simulink model "AGTF30SysDyn_PExPIn"  (R2023b)
settings: Solver=ode4  StartTime=0.0  StopTime=MWS.In.tend  FixedStep=MWS.In.Ts  RelTol=1e-3  EnableMultiTasking=on
model workspace: external: MAT-File (data not in the file)
values from neighbouring files (symbols this model uses):
  MWS = setup_initialize(MWS,startPt,SSsolverSP)    [Setup_Simulation.m]    (also in run_AGTF30e_script.m = Setup_Simulation(inputMethod,MWS.In,filename,Mdl,SSsolverSP))
undefined symbols (not defined in the file or in its folder): DiscIntNeverNeededParam
libraries: simulink x32, Lib_Solve_ModelSource_TMATS x28, Lib_EMTAT x27, Lib_Cntrl_FirstOrderSensor_TMATS x19, Lib_Cntrl_FirstOrderActuator_TMATS x2, Lib_Cntrl_LimitSelect_TMATS x2, Lib_Solve_OuterLoopIntegrator_TMATS x2, Lib_Cntrl_CorrectedSpeed_TMATS x1, Lib_Solve_IterNRSolverJC_TMATS x1, slpidlib x1
(part 2 of 8)

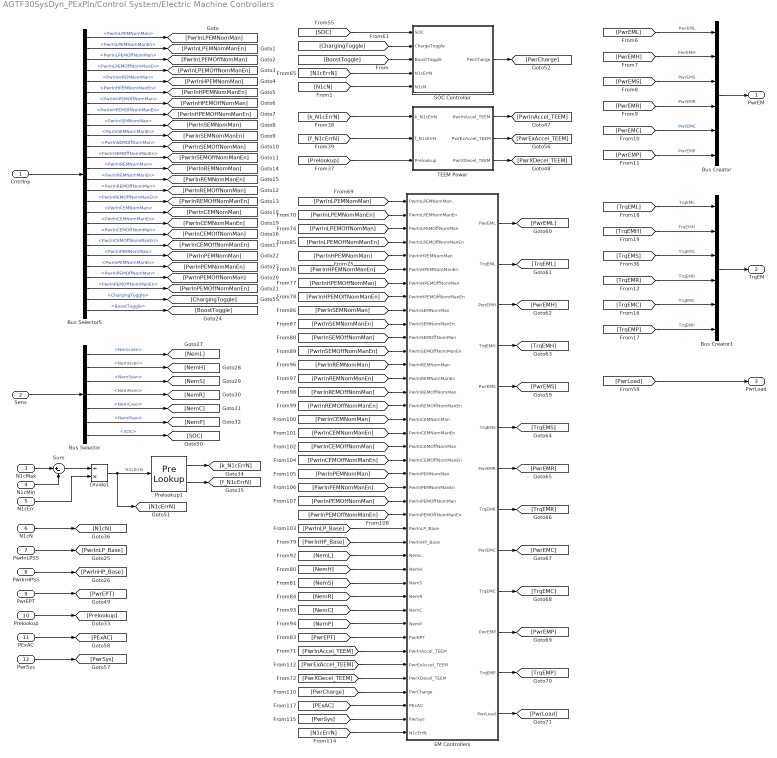
== system AGTF30SysDyn_PExPIn/Control System/Electric Machine Controllers ==
  CntrlInp : Inport
  Sens : Inport  Port=2
  N1cMax : Inport  Port=3
  N1cMin : Inport  Port=4
  N1cErr : Inport  Port=5
  N1cN : Inport  Port=6
  PwrInLPSS : Inport  Port=7
  PwrInHPSS : Inport  Port=8
  PwrEPT : Inport  Port=9
  Prelookup : Inport  Port=10
  PExAC : Inport  Port=11
  PwrSys : Inport  Port=12
  Bus Creator : BusCreator  Inputs=6
  Bus Creator1 : BusCreator  Inputs=6
  Bus Selector : BusSelector  OutputSignals=N.NemLsen,N.NemHsen,N.NemSsen,N.NemRsen,N.NemCsen,N.NemPsen,SOC
  Bus Selector5 : BusSelector  OutputSignals=ManualOp.PwrInLPEMNomMan,ManualOp.PwrInLPEMNomManEn,ManualOp.PwrInLPEMOffNomMan,ManualOp.PwrInLPEMOffNomManEn,ManualOp.PwrInHPEMNomMan,ManualOp.PwrInHPEMNomManEn,ManualOp.PwrInHPEMOffNomMan,ManualOp.PwrInHPEMOffNomManEn,ManualOp.PwrInSEMNomMan,ManualOp.PwrInSEMNomManEn,ManualOp.PwrInSEMOffNomMan,ManualOp.PwrInSEMOffNomManEn,ManualOp.PwrInREMNomMan,ManualOp.PwrInREMNomManEn,ManualOp.PwrInREMOffNomMan,ManualOp.PwrInREMOffNomManEn,ManualOp.PwrInCEMNomMan,ManualOp.PwrInCEMNomManEn,ManualOp.PwrInCEMOffNomMan,ManualOp.PwrInCEMOffNomManEn,ManualOp.PwrInPEMNomMan,ManualOp.PwrInPEMNomManEn,ManualOp.PwrInPEMOffNomMan,ManualOp.PwrInPEMOffNomManEn,PilotCmd.ChargingToggle,PilotCmd.BoostToggle
  Divide1 : Product  Inputs=/*
  EM Controllers : Subsystem  Variant=on
  Prelookup1 : PreLookup  BreakpointsData=MWS.Cntrl.TEEM.N1cErrN_vec  ExtrapMethod=Linear
  SOC Controller : Subsystem
  Sum : Sum  Inputs=|+-
  TEEM Power : Subsystem
  PwrEM : Outport
  TrqEM : Outport  Port=2
  PwrLoad : Outport  Port=3
  wires:
  Bus Selector5/19 -> [PwrInCEMOffNomMan]  "<PwrInCEMOffNomMan>"
  Sum/1 -> Divide1/1
  Bus Selector5/10 -> [PwrInSEMNomManEn]  "<PwrInSEMNomManEn>"
  Bus Selector5/4 -> [PwrInLPEMOffNomManEn]  "<PwrInLPEMOffNomManEn>"
  Bus Selector5/13 -> [PwrInREMNomMan]  "<PwrInREMNomMan>"
  Bus Selector5/24 -> [PwrInPEMOffNomManEn]  "<PwrInPEMOffNomManEn>"
  Bus Selector5/18 -> [PwrInCEMNomManEn]  "<PwrInCEMNomManEn>"
  Bus Selector5/20 -> [PwrInCEMOffNomManEn]  "<PwrInCEMOffNomManEn>"
  Bus Selector5/15 -> [PwrInREMOffNomMan]  "<PwrInREMOffNomMan>"
  Bus Selector5/17 -> [PwrInCEMNomMan]  "<PwrInCEMNomMan>"
  Bus Selector5/1 -> [PwrInLPEMNomMan]  "<PwrInLPEMNomMan>"
  Bus Selector5/21 -> [PwrInPEMNomMan]  "<PwrInPEMNomMan>"
  Bus Selector5/23 -> [PwrInPEMOffNomMan]  "<PwrInPEMOffNomMan>"
  Bus Selector5/11 -> [PwrInSEMOffNomMan]  "<PwrInSEMOffNomMan>"
  Bus Selector5/22 -> [PwrInPEMNomManEn]  "<PwrInPEMNomManEn>"
  N1cErr/1 -> Divide1/2
  Bus Selector5/6 -> [PwrInHPEMNomManEn]  "<PwrInHPEMNomManEn>"
  PwrInLPSS/1 -> [PwrInLP_Base]
  N1cMax/1 -> Sum/1
  Bus Selector5/9 -> [PwrInSEMNomMan]  "<PwrInSEMNomMan>"
  Bus Selector5/7 -> [PwrInHPEMOffNomMan]  "<PwrInHPEMOffNomMan>"
  Bus Selector5/8 -> [PwrInHPEMOffNomManEn]  "<PwrInHPEMOffNomManEn>"
  Bus Selector5/5 -> [PwrInHPEMNomMan]  "<PwrInHPEMNomMan>"
  Bus Selector5/3 -> [PwrInLPEMOffNomMan]  "<PwrInLPEMOffNomMan>"
  Bus Selector5/14 -> [PwrInREMNomManEn]  "<PwrInREMNomManEn>"
  Bus Selector5/12 -> [PwrInSEMOffNomManEn]  "<PwrInSEMOffNomManEn>"
  Bus Selector5/16 -> [PwrInREMOffNomManEn]  "<PwrInREMOffNomManEn>"
  CntrlInp/1 -> Bus Selector5/1
  Bus Selector5/2 -> [PwrInLPEMNomManEn]  "<PwrInLPEMNomManEn>"
  N1cMin/1 -> Sum/2
  Divide1/1 -> [N1cErrN], Prelookup1/1  "N1cErrN"
  PwrInHPSS/1 -> [PwrInHP_Base]
  Sens/1 -> Bus Selector/1
  Bus Selector/1 -> [NemL]  "<NemLsen>"
  Bus Selector/2 -> [NemH]  "<NemHsen>"
  Bus Selector/3 -> [NemS]  "<NemSsen>"
  Bus Selector/4 -> [NemR]  "<NemRsen>"
  Bus Selector/5 -> [NemC]  "<NemCsen>"
  Bus Selector/6 -> [NemP]  "<NemPsen>"
  Bus Creator/1 -> PwrEM/1
  [PwrEML] -> Bus Creator/1  "PwrEML"
  [PwrEMH] -> Bus Creator/2  "PwrEMH"
  [PwrEMS] -> Bus Creator/3  "PwrEMS"
  [PwrEMR] -> Bus Creator/4  "PwrEMR"
  [PwrEMC] -> Bus Creator/5  "PwrEMC"
  [PwrEMP] -> Bus Creator/6  "PwrEMP"
  Bus Creator1/1 -> TrqEM/1
  [TrqEML] -> Bus Creator1/1  "TrqEML"
  [TrqEMH] -> Bus Creator1/2  "TrqEMH"
  [TrqEMS] -> Bus Creator1/3  "TrqEMS"
  [TrqEMR] -> Bus Creator1/4  "TrqEMR"
  [TrqEMC] -> Bus Creator1/5  "TrqEMC"
  [TrqEMP] -> Bus Creator1/6  "TrqEMP"
  Prelookup/1 -> [Prelookup]
  Prelookup1/1 -> [k_N1cErrN]
  Prelookup1/2 -> [f_N1cErrN]
  [k_N1cErrN] -> TEEM Power/1(k_N1cErrN)
  [f_N1cErrN] -> TEEM Power/2(f_N1cErrN)
  [Prelookup] -> TEEM Power/3(Prelookup)
  TEEM Power/1(PwrInAccel_TEEM) -> [PwrInAccel_TEEM]
  TEEM Power/3(PwrXDecel_TEEM) -> [PwrXDecel_TEEM]
  PwrEPT/1 -> [PwrEPT]
  Bus Selector/7 -> [SOC]  "<SOC>"
  [SOC] -> SOC Controller/1(SOC)
  SOC Controller/1(PwrCharge) -> [PwrCharge]
  [PwrLoad] -> PwrLoad/1
  Bus Selector5/25 -> [ChargingToggle]  "<ChargingToggle>"
  [ChargingToggle] -> SOC Controller/2(ChargeToggle)
  TEEM Power/2(PwrExAccel_TEEM) -> [PwrExAccel_TEEM]
  PwrSys/1 -> [PwrSys]
  [N1cErrN] -> SOC Controller/4(N1cErrN)
  PExAC/1 -> [PExAC]
  [PwrInLPEMNomMan] -> EM Controllers/1(PwrInLPEMNomMan)
  [PwrInLPEMNomManEn] -> EM Controllers/2(PwrInLPEMNomManEn)
  [PwrInLPEMOffNomMan] -> EM Controllers/3(PwrInLPEMOffNomMan)
  [PwrInLPEMOffNomManEn] -> EM Controllers/4(PwrInLPEMOffNomManEn)
  [PwrInHPEMNomMan] -> EM Controllers/5(PwrInHPEMNomMan)
  [PwrInHPEMNomManEn] -> EM Controllers/6(PwrInHPEMNomManEn)
  [PwrInHPEMOffNomMan] -> EM Controllers/7(PwrInHPEMOffNomMan)
  [PwrInHPEMOffNomManEn] -> EM Controllers/8(PwrInHPEMOffNomManEn)
  [PwrInSEMNomMan] -> EM Controllers/9(PwrInSEMNomMan)
  [PwrInSEMNomManEn] -> EM Controllers/10(PwrInSEMNomManEn)
  [PwrInSEMOffNomMan] -> EM Controllers/11(PwrInSEMOffNomMan)
  [PwrInSEMOffNomManEn] -> EM Controllers/12(PwrInSEMOffNomManEn)
  [PwrInREMNomMan] -> EM Controllers/13(PwrInREMNomMan)
  [PwrInREMNomManEn] -> EM Controllers/14(PwrInREMNomManEn)
  [PwrInREMOffNomMan] -> EM Controllers/15(PwrInREMOffNomMan)
  [PwrInREMOffNomManEn] -> EM Controllers/16(PwrInREMOffNomManEn)
  [PwrInCEMNomMan] -> EM Controllers/17(PwrInCEMNomMan)
  [PwrInCEMNomManEn] -> EM Controllers/18(PwrInCEMNomManEn)
  [PwrInCEMOffNomMan] -> EM Controllers/19(PwrInCEMOffNomMan)
  [PwrInCEMOffNomManEn] -> EM Controllers/20(PwrInCEMOffNomManEn)
  [PwrInPEMNomMan] -> EM Controllers/21(PwrInPEMNomMan)
  [PwrInPEMNomManEn] -> EM Controllers/22(PwrInPEMNomManEn)
  [PwrInPEMOffNomMan] -> EM Controllers/23(PwrInPEMOffNomMan)
  [PwrInPEMOffNomManEn] -> EM Controllers/24(PwrInPEMOffNomManEn)
  [PwrInLP_Base] -> EM Controllers/25(PwrInLP_Base)
  [PwrInHP_Base] -> EM Controllers/26(PwrInHP_Base)
  [NemL] -> EM Controllers/27(NemL)
  [NemH] -> EM Controllers/28(NemH)
  [NemS] -> EM Controllers/29(NemS)
  [NemR] -> EM Controllers/30(NemR)
  [NemC] -> EM Controllers/31(NemC)
  [NemP] -> EM Controllers/32(NemP)
  [PwrEPT] -> EM Controllers/33(PwrEPT)
  [PwrInAccel_TEEM] -> EM Controllers/34(PwrInAccel_TEEM)
  [PwrExAccel_TEEM] -> EM Controllers/35(PwrExAccel_TEEM)
  [PwrXDecel_TEEM] -> EM Controllers/36(PwrXDecel_TEEM)
  [PwrCharge] -> EM Controllers/37(PwrCharge)
  [PExAC] -> EM Controllers/38(PExAC)
  [PwrSys] -> EM Controllers/39(PwrSys)
  [N1cErrN] -> EM Controllers/40(N1cErrN)
  EM Controllers/13(PwrLoad) -> [PwrLoad]
  EM Controllers/1(PwrEML) -> [PwrEML]
  EM Controllers/3(PwrEMH) -> [PwrEMH]
  EM Controllers/2(TrqEML) -> [TrqEML]
  EM Controllers/4(TrqEMH) -> [TrqEMH]
  EM Controllers/12(TrqEMP) -> [TrqEMP]
  EM Controllers/11(PwrEMP) -> [PwrEMP]
  EM Controllers/10(TrqEMC) -> [TrqEMC]
  EM Controllers/9(PwrEMC) -> [PwrEMC]
  EM Controllers/8(TrqEMR) -> [TrqEMR]
  EM Controllers/7(PwrEMR) -> [PwrEMR]
  EM Controllers/6(TrqEMS) -> [TrqEMS]
  EM Controllers/5(PwrEMS) -> [PwrEMS]
  Bus Selector5/26 -> [BoostToggle]  "<BoostToggle>"
  [BoostToggle] -> SOC Controller/3(BoostToggle)
  N1cN/1 -> [N1cN]
  [N1cN] -> SOC Controller/5(N1cN)

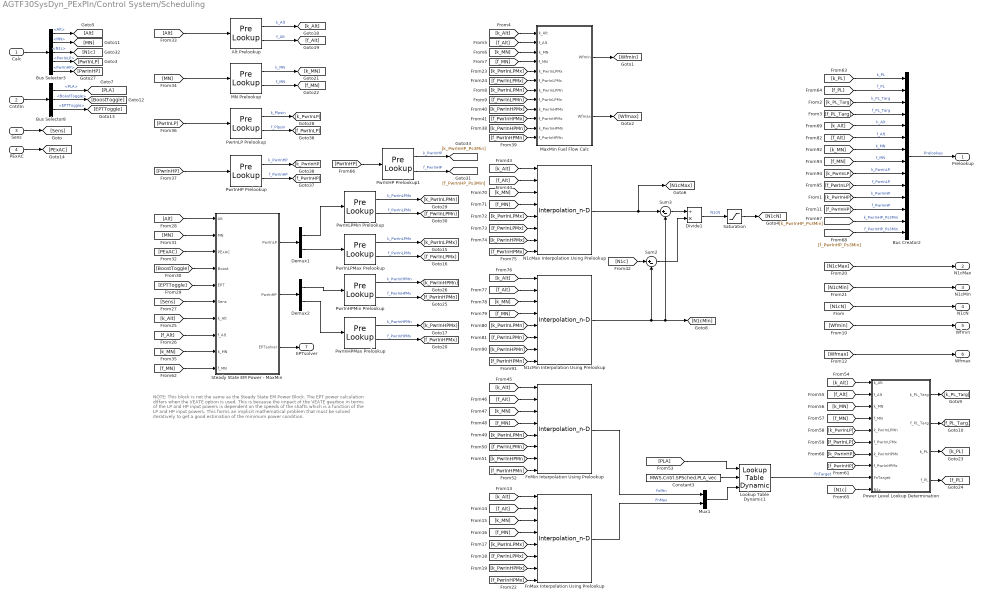
== system AGTF30SysDyn_PExPIn/Control System/Scheduling ==
  note: NOTE: This block is not the same as the Steady State EM Power Block. The EPT power calculation differs when the VEATE option is used. This is because the impact of the VEATE gearbox in terms of the LP and HP input powers is dependent on the speeds of the shafts which is a function of the LP and HP input powers. This forms an implicit mathematical problem that must be solved iteratively to get a good estimation of the minimum power condition.
  Calc : Inport
  CntrlIn : Inport  Port=2
  Sens : Inport  Port=3
  PExAC : Inport  Port=4
  Alt Prelookup : PreLookup  BreakpointsData=MWS.Cntrl.SPSched.Alt_vec  IndexSearchMethod=Linear search  BeginIndexSearchUsingPreviousIndexResult=on
  Bus Creator2 : BusCreator  Inputs=14
  Bus Selector3 : BusSelector  OutputSignals=Alt,MN,N1c,PwrInLP,PwrInHP
  Bus Selector8 : BusSelector  OutputSignals=PilotCmd.PLA,PilotCmd.BoostToggle,PilotCmd.EPTToggle
  Constant3 : Constant  Value=MWS.Cntrl.SPSched.PLA_vec
  Demux1 : Demux  Outputs=2
  Demux2 : Demux  Outputs=2
  Divide1 : Product  Inputs=/*
  FnMax Interpolation Using Prelookup : Interpolation_n-D  NumberOfTableDimensions=4  Table=MWS.Cntrl.Sched.FnMax.FnMax_array  DiagnosticForOutOfRangeInput=Error  InternalRulePriority=Speed
      settings: InputPortMap=u0,u1,u2,u3,u4,u5,u6,u7
  FnMin Interpolation Using Prelookup : Interpolation_n-D  NumberOfTableDimensions=4  Table=MWS.Cntrl.Sched.FnMin.FnMin_array  DiagnosticForOutOfRangeInput=Error  InternalRulePriority=Speed
      settings: InputPortMap=u0,u1,u2,u3,u4,u5,u6,u7
  Lookup Table Dynamic1 : simulink/Lookup Tables/Lookup Table Dynamic  LookUpMeth=Interpolation-Use End Values  OutDataType=fixdt('double')  OutScaling=[]  OutputDataTypeScalingMode=Specify via dialog  OutDataTypeStr=double  DoSatur=off
  MN Prelookup : PreLookup  BreakpointsData=MWS.Cntrl.SPSched.MN_vec  IndexSearchMethod=Linear search  BeginIndexSearchUsingPreviousIndexResult=on
  MaxMin Fuel Flow Calc : Subsystem
  Mux1 : Mux  Inputs=2
  N1cMax Interpolation Using Prelookup : Interpolation_n-D  NumberOfTableDimensions=4  Table=MWS.Cntrl.Sched.N1cMax.N1cMax_array  DiagnosticForOutOfRangeInput=Error  InternalRulePriority=Speed
      settings: InputPortMap=u0,u1,u2,u3,u4,u5,u6,u7
  N1cMin Interpolation Using Prelookup : Interpolation_n-D  NumberOfTableDimensions=4  Table=MWS.Cntrl.Sched.N1cMin.N1cMin_array  DiagnosticForOutOfRangeInput=Error  InternalRulePriority=Speed
      settings: InputPortMap=u0,u1,u2,u3,u4,u5,u6,u7
  Power Level Lookup Determination : Subsystem
  PwrInHP Prelookup : PreLookup  BreakpointsData=MWS.Cntrl.SPSched.PwrInHP_vec  IndexSearchMethod=Linear search  BeginIndexSearchUsingPreviousIndexResult=on
  PwrInHP Prelookup1 : PreLookup  BreakpointsData=MWS.Cntrl.WfCntrl.Ps3Min.PwrInHP_vec  IndexSearchMethod=Linear search  BeginIndexSearchUsingPreviousIndexResult=on
  PwrInHPMax Prelookup : PreLookup  BreakpointsData=MWS.Cntrl.SPSched.PwrInHP_vec  IndexSearchMethod=Linear search  BeginIndexSearchUsingPreviousIndexResult=on
  PwrInHPMin Prelookup : PreLookup  BreakpointsData=MWS.Cntrl.SPSched.PwrInHP_vec  IndexSearchMethod=Linear search  BeginIndexSearchUsingPreviousIndexResult=on
  PwrInLP Prelookup : PreLookup  BreakpointsData=MWS.Cntrl.SPSched.PwrInLP_vec  IndexSearchMethod=Linear search  BeginIndexSearchUsingPreviousIndexResult=on
  PwrInLPMax Prelookup : PreLookup  BreakpointsData=MWS.Cntrl.SPSched.PwrInLP_vec  IndexSearchMethod=Linear search  BeginIndexSearchUsingPreviousIndexResult=on
  PwrInLPMin Prelookup : PreLookup  BreakpointsData=MWS.Cntrl.SPSched.PwrInLP_vec  IndexSearchMethod=Linear search  BeginIndexSearchUsingPreviousIndexResult=on
  Saturation : Saturate  UpperLimit=1  LowerLimit=0
  Steady State EM Power - MaxMin : Subsystem
  Sum2 : Sum  Inputs=|+-
  Sum3 : Sum  Inputs=|+-
  Prelookup : Outport
  N1cMax : Outport  Port=2
  N1cMin : Outport  Port=3
  N1cN : Outport  Port=4
  Wfmin : Outport  Port=5
  Wfmax : Outport  Port=6
  EPTsolver : Outport  Port=7
  wires:
  [k_Alt] -> Bus Creator2/5  "k_Alt"
  [MN] -> MN Prelookup/1
  Alt Prelookup/2 -> [f_Alt]  "f_Alt"
  PwrInLPMin Prelookup/1 -> [k_PwrInLPMn]  "k_PwrInLPMn"
  [f_PwrInLP] -> Bus Creator2/10  "f_PwrInLP"
  [Alt] -> Alt Prelookup/1
  PwrInLPMin Prelookup/2 -> [f_PwrInLPMn]  "f_PwrInLPMx"
  [k_MN] -> Bus Creator2/7  "k_MN"
  MN Prelookup/1 -> [k_MN]  "k_MN"
  [k_PwrInLP] -> Bus Creator2/9  "k_PwrInLP"
  MN Prelookup/2 -> [f_MN]  "f_MN"
  Alt Prelookup/1 -> [k_Alt]  "k_Alt"
  [k_PL_Targ] -> Bus Creator2/3  "k_PL_Targ"
  [f_PL_Targ] -> Bus Creator2/4  "f_PL_Targ"
  [f_Alt] -> Bus Creator2/6  "f_Alt"
  [f_MN] -> Bus Creator2/8  "f_MN"
  Bus Creator2/1 -> Prelookup/1  "Prelookup"
  [Wfmin] -> Wfmin/1
  [Wfmax] -> Wfmax/1
  Sens/1 -> [Sens]
  Calc/1 -> Bus Selector3/1
  Bus Selector3/1 -> [Alt]  "<Alt>"
  Bus Selector3/2 -> [MN]  "<MN>"
  CntrlIn/1 -> Bus Selector8/1
  Bus Selector8/2 -> [BoostToggle]  "<BoostToggle>"
  Bus Selector8/3 -> [EPTToggle]  "<EPTToggle>"
  [EPTToggle] -> Steady State EM Power - MaxMin/5(EPT)
  [BoostToggle] -> Steady State EM Power - MaxMin/4(Boost)
  [Alt] -> Steady State EM Power - MaxMin/1(Alt)
  [MN] -> Steady State EM Power - MaxMin/2(MN)
  PExAC/1 -> [PExAC]
  [PExAC] -> Steady State EM Power - MaxMin/3(PExAC)
  Steady State EM Power - MaxMin/1(PwrInLP) -> Demux1/1
  Steady State EM Power - MaxMin/2(PwrInHP) -> Demux2/1
  Demux1/2 -> PwrInLPMax Prelookup/1
  Demux1/1 -> PwrInLPMin Prelookup/1
  PwrInLPMax Prelookup/1 -> [k_PwrInLPMx]  "k_PwrInLPMn"
  PwrInLPMax Prelookup/2 -> [f_PwrInLPMx]  "f_PwrInLPMx"
  PwrInHPMax Prelookup/2 -> [f_PwrInHPMx]  "f_PwrInHPMx"
  PwrInHPMax Prelookup/1 -> [k_PwrInHPMx]  "k_PwrInHPMn"
  PwrInHPMin Prelookup/2 -> [f_PwrInHPMn]  "f_PwrInHPMx"
  Demux2/1 -> PwrInHPMin Prelookup/1
  Demux2/2 -> PwrInHPMax Prelookup/1
  PwrInHPMin Prelookup/1 -> [k_PwrInHPMn]  "k_PwrInHPMn"
  Bus Selector3/3 -> [N1c]  "<N1c>"
  [PwrInLP] -> PwrInLP Prelookup/1
  PwrInLP Prelookup/1 -> [k_PwrInLP]  "k_Plpsin"
  PwrInLP Prelookup/2 -> [f_PwrInLP]  "f_Plpsin"
  PwrInHP Prelookup/1 -> [k_PwrInHP]  "k_PwrInHP"
  PwrInHP Prelookup/2 -> [f_PwrInHP]  "f_PwrInHP"
  [PwrInHP] -> PwrInHP Prelookup/1
  [k_Alt] -> MaxMin Fuel Flow Calc/1(k_Alt)
  [f_Alt] -> MaxMin Fuel Flow Calc/2(f_Alt)
  [k_MN] -> MaxMin Fuel Flow Calc/3(k_MN)
  [f_MN] -> MaxMin Fuel Flow Calc/4(f_MN)
  [k_PwrInLPMn] -> MaxMin Fuel Flow Calc/7(k_PwrInLPMn)
  [f_PwrInLPMn] -> MaxMin Fuel Flow Calc/8(f_PwrInLPMn)
  [f_PwrInLPMx] -> MaxMin Fuel Flow Calc/6(f_PwrInLPMx)
  [k_PwrInLPMx] -> MaxMin Fuel Flow Calc/5(k_PwrInLPMx)
  [k_PwrInHPMn] -> MaxMin Fuel Flow Calc/11(k_PwrInHPMn)
  [f_PwrInHPMn] -> MaxMin Fuel Flow Calc/12(f_PwrInHPMn)
  [k_PwrInHPMx] -> MaxMin Fuel Flow Calc/9(k_PwrInHPMx)
  [f_PwrInHPMx] -> MaxMin Fuel Flow Calc/10(f_PwrInHPMx)
  MaxMin Fuel Flow Calc/1(Wfmin) -> [Wfmin]
  MaxMin Fuel Flow Calc/2(Wfmax) -> [Wfmax]
  [k_Alt] -> N1cMax Interpolation Using Prelookup/1
  [f_Alt] -> N1cMax Interpolation Using Prelookup/2
  [k_MN] -> N1cMax Interpolation Using Prelookup/3
  [f_MN] -> N1cMax Interpolation Using Prelookup/4
  [k_PwrInHPMx] -> N1cMax Interpolation Using Prelookup/7
  [f_PwrInLPMx] -> N1cMax Interpolation Using Prelookup/6
  [k_PwrInLPMx] -> N1cMax Interpolation Using Prelookup/5
  [f_PwrInHPMx] -> N1cMax Interpolation Using Prelookup/8
  [f_PwrInHPMn] -> N1cMin Interpolation Using Prelookup/8
  [k_PwrInLPMn] -> N1cMin Interpolation Using Prelookup/5
  [f_PwrInLPMn] -> N1cMin Interpolation Using Prelookup/6
  [k_PwrInHPMn] -> N1cMin Interpolation Using Prelookup/7
  [f_MN] -> N1cMin Interpolation Using Prelookup/4
  [k_MN] -> N1cMin Interpolation Using Prelookup/3
  [f_Alt] -> N1cMin Interpolation Using Prelookup/2
  [k_Alt] -> N1cMin Interpolation Using Prelookup/1
  [N1c] -> Sum2/1
  N1cMax Interpolation Using Prelookup/1 -> [N1cMax], Sum3/1
  Sum3/1 -> Divide1/1
  Sum2/1 -> Divide1/2
  N1cMin Interpolation Using Prelookup/1 -> [N1cMin], Sum3/2, Sum2/2
  Divide1/1 -> Saturation/1  "N1cN"
  [k_Alt] -> FnMin Interpolation Using Prelookup/1
  [f_Alt] -> FnMin Interpolation Using Prelookup/2
  [k_MN] -> FnMin Interpolation Using Prelookup/3
  [f_MN] -> FnMin Interpolation Using Prelookup/4
  [k_PwrInHPMn] -> FnMin Interpolation Using Prelookup/7
  [f_PwrInLPMn] -> FnMin Interpolation Using Prelookup/6
  [k_PwrInLPMn] -> FnMin Interpolation Using Prelookup/5
  [f_PwrInHPMn] -> FnMin Interpolation Using Prelookup/8
  [f_PwrInHPMx] -> FnMax Interpolation Using Prelookup/8
  [k_PwrInLPMx] -> FnMax Interpolation Using Prelookup/5
  [f_PwrInLPMx] -> FnMax Interpolation Using Prelookup/6
  [k_PwrInHPMx] -> FnMax Interpolation Using Prelookup/7
  [f_MN] -> FnMax Interpolation Using Prelookup/4
  [k_MN] -> FnMax Interpolation Using Prelookup/3
  [f_Alt] -> FnMax Interpolation Using Prelookup/2
  [k_Alt] -> FnMax Interpolation Using Prelookup/1
  FnMax Interpolation Using Prelookup/1 -> Mux1/2  "FnMax"
  FnMin Interpolation Using Prelookup/1 -> Mux1/1  "FnMin"
  Bus Selector8/1 -> [PLA]  "<PLA>"
  [PLA] -> Lookup Table Dynamic1/1
  Constant3/1 -> Lookup Table Dynamic1/2
  Mux1/1 -> Lookup Table Dynamic1/3
  Lookup Table Dynamic1/1 -> Power Level Lookup Determination/9(FnTarget)  "FnTarget"
  Power Level Lookup Determination/2(f_PL_Targ) -> [f_PL_Targ]
  Power Level Lookup Determination/1(k_PL_Targ) -> [k_PL_Targ]
  [k_PwrInHP] -> Bus Creator2/11  "k_PwrInHP"
  [f_PwrInHP] -> Bus Creator2/12  "f_PwrInHP"
  [N1cN] -> N1cN/1
  [Sens] -> Steady State EM Power - MaxMin/6(Sens)
  Bus Selector3/4 -> [PwrInLP]  "<PwrInLP>"
  Bus Selector3/5 -> [PwrInHP]  "<PwrInHP>"
  [N1cMin] -> N1cMin/1
  [N1cMax] -> N1cMax/1
  [k_Alt] -> Steady State EM Power - MaxMin/7(k_Alt)
  [f_Alt] -> Steady State EM Power - MaxMin/8(f_Alt)
  [k_MN] -> Steady State EM Power - MaxMin/9(k_MN)
  [f_MN] -> Steady State EM Power - MaxMin/10(f_MN)
  Steady State EM Power - MaxMin/3(EPTsolver) -> EPTsolver/1
  Saturation/1 -> [N1cN]
  [k_Alt] -> Power Level Lookup Determination/1(k_Alt)
  [f_Alt] -> Power Level Lookup Determination/2(f_Alt)
  [k_MN] -> Power Level Lookup Determination/3(k_MN)
  [f_MN] -> Power Level Lookup Determination/4(f_MN)
  [k_PwrInLP] -> Power Level Lookup Determination/5(k_PwrInLPMn)
  [f_PwrInLP] -> Power Level Lookup Determination/6(f_PwrInLPMx)
  [k_PwrInHP] -> Power Level Lookup Determination/7(k_PwrInHPMn)
  [f_PwrInHP] -> Power Level Lookup Determination/8(f_PwrInHPMx)
  [k_PL] -> Bus Creator2/1  "k_PL"
  [f_PL] -> Bus Creator2/2  "f_PL"
  [N1c] -> Power Level Lookup Determination/10(N1c)
  Power Level Lookup Determination/3(k_PL) -> [k_PL]
  Power Level Lookup Determination/4(f_PL) -> [f_PL]
  PwrInHP Prelookup1/1 -> [k_PwrInHP_Ps3Min]  "k_PwrInHP"
  PwrInHP Prelookup1/2 -> [f_PwrInHP_Ps3Min]  "f_PwrInHP"
  [PwrInHP] -> PwrInHP Prelookup1/1
  [k_PwrInHP_Ps3Min] -> Bus Creator2/13  "k_PwrInHP_Ps3Min"
  [f_PwrInHP_Ps3Min] -> Bus Creator2/14  "f_PwrInHP_Ps3Min"

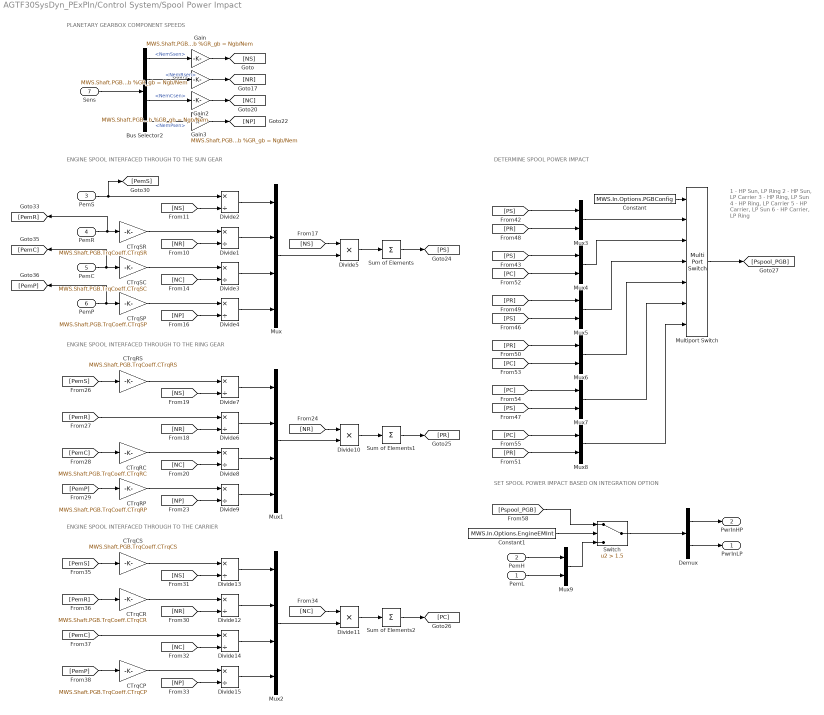
== system AGTF30SysDyn_PExPIn/Control System/Spool Power Impact ==
  note: 1 - HP Sun, LP Ring
      | 2 - HP Sun, LP Carrier
      | 3 - HP Ring, LP Sun
      | 4 - HP Ring, LP Carrier
      | 5 - HP Carrier, LP Sun
      | 6 - HP Carrier, LP Ring
  note: ENGINE SPOOL INTERFACED THROUGH TO THE SUN GEAR
  note: ENGINE SPOOL INTERFACED THROUGH TO THE RING GEAR
  note: ENGINE SPOOL INTERFACED THROUGH TO THE CARRIER
  note: DETERMINE SPOOL POWER IMPACT
  note: SET SPOOL POWER IMPACT BASED ON INTEGRATION OPTION
  note: PLANETARY GEARBOX COMPONENT SPEEDS
  PemL : Inport
  PemH : Inport  Port=2
  PemS : Inport  Port=3
  PemR : Inport  Port=4
  PemC : Inport  Port=5
  PemP : Inport  Port=6
  Sens : Inport  Port=7
  Bus Selector2 : BusSelector  OutputSignals=N.NemSsen,N.NemRsen,N.NemCsen,N.NemPsen
  CTrqCP : Gain  Gain=MWS.Shaft.PGB.TrqCoeff.CTrqCP
  CTrqCR : Gain  Gain=MWS.Shaft.PGB.TrqCoeff.CTrqCR
  CTrqCS : Gain  Gain=MWS.Shaft.PGB.TrqCoeff.CTrqCS
  CTrqRC : Gain  Gain=MWS.Shaft.PGB.TrqCoeff.CTrqRC
  CTrqRP : Gain  Gain=MWS.Shaft.PGB.TrqCoeff.CTrqRP
  CTrqRS : Gain  Gain=MWS.Shaft.PGB.TrqCoeff.CTrqRS
  CTrqSC : Gain  Gain=MWS.Shaft.PGB.TrqCoeff.CTrqSC
  CTrqSP : Gain  Gain=MWS.Shaft.PGB.TrqCoeff.CTrqSP
  CTrqSR : Gain  Gain=MWS.Shaft.PGB.TrqCoeff.CTrqSR
  Constant : Constant  Value=MWS.In.Options.PGBConfig
  Constant1 : Constant  Value=MWS.In.Options.EngineEMInt
  Demux : Demux  Outputs=2
  Divide{1..4,6..9,12..15} (12 alike) : Product  Inputs=*/
  Divide10 : Product  Inputs=**
  Divide11 : Product  Inputs=**
  Divide5 : Product  Inputs=**
  Gain : Gain  Gain=MWS.Shaft.PGB.Sun.GR_gb %GR_gb = Ngb/Nem
  Gain1 : Gain  Gain=MWS.Shaft.PGB.Ring.GR_gb %GR_gb = Ngb/Nem
  Gain2 : Gain  Gain=MWS.Shaft.PGB.Carrier.GR_gb %GR_gb = Ngb/Nem
  Gain3 : Gain  Gain=MWS.Shaft.PGB.Planet.GR_gb %GR_gb = Ngb/Nem
  Multiport Switch : MultiPortSwitch  Inputs=6  SaturateOnIntegerOverflow=off  InputSameDT=off
  Mux : Mux
  Mux1 : Mux
  Mux2 : Mux
  Mux{3..9} (7 alike) : Mux  Inputs=2
  Sum of Elements : Sum  Inputs=+
  Sum of Elements1 : Sum  Inputs=+
  Sum of Elements2 : Sum  Inputs=+
  Switch : Switch  Criteria=u2 > Threshold  Threshold=1.5  SaturateOnIntegerOverflow=off  InputSameDT=off
  PwrInLP : Outport
  PwrInHP : Outport  Port=2
  wires:
  [PemP] -> CTrqRP/1
  CTrqRC/1 -> Divide8/1
  [NP] -> Divide4/2
  CTrqRP/1 -> Divide9/1
  [PemS] -> CTrqCS/1
  Mux8/1 -> Multiport Switch/7
  [NC] -> Divide14/2
  Mux5/1 -> Multiport Switch/4
  [PR] -> Mux5/1
  [NP] -> Divide15/2
  CTrqCS/1 -> Divide13/1
  CTrqCP/1 -> Divide15/1
  [PR] -> Mux3/2
  [PC] -> Mux8/1
  CTrqRS/1 -> Divide7/1
  Divide4/1 -> Mux/4
  [PS] -> Mux5/2
  Switch/1 -> Demux/1
  [NS] -> Divide7/2
  [PR] -> Mux8/2
  Constant1/1 -> Switch/2
  Divide11/1 -> Sum of Elements2/1
  Divide7/1 -> Mux1/1
  CTrqSR/1 -> Divide1/1
  Divide14/1 -> Mux2/3
  [PemC] -> Divide14/1
  [PemC] -> CTrqRC/1
  Mux4/1 -> Multiport Switch/3
  [PC] -> Mux4/2
  [NP] -> Divide9/2
  CTrqSC/1 -> Divide3/1
  Divide2/1 -> Mux/1
  Mux2/1 -> Divide11/2
  PemR/1 -> [PemR], CTrqSR/1
  [NR] -> Divide12/2
  Divide15/1 -> Mux2/4
  Divide8/1 -> Mux1/3
  [NS] -> Divide2/2
  [PC] -> Mux6/2
  Constant/1 -> Multiport Switch/1
  [PemP] -> CTrqCP/1
  Divide10/1 -> Sum of Elements1/1
  [NC] -> Divide11/1
  Divide3/1 -> Mux/3
  [NS] -> Divide5/1
  Divide13/1 -> Mux2/1
  [NS] -> Divide13/2
  [NR] -> Divide1/2
  Mux6/1 -> Multiport Switch/5
  Divide5/1 -> Sum of Elements/1
  Divide12/1 -> Mux2/2
  PemP/1 -> [PemP], CTrqSP/1
  [PS] -> Mux3/1
  [NR] -> Divide10/1
  [PR] -> Mux6/1
  PemS/1 -> [PemS], Divide2/1
  [PemS] -> CTrqRS/1
  [NC] -> Divide3/2
  CTrqSP/1 -> Divide4/1
  Mux7/1 -> Multiport Switch/6
  [Pspool_PGB] -> Switch/1
  CTrqCR/1 -> Divide12/1
  Mux9/1 -> Switch/3
  Divide1/1 -> Mux/2
  [PemR] -> CTrqCR/1
  PemC/1 -> [PemC], CTrqSC/1
  [PC] -> Mux7/1
  [PS] -> Mux7/2
  [PS] -> Mux4/1
  Multiport Switch/1 -> [Pspool_PGB]
  [PemR] -> Divide6/1
  Mux3/1 -> Multiport Switch/2
  [NC] -> Divide8/2
  Divide9/1 -> Mux1/4
  Mux1/1 -> Divide10/2
  Divide6/1 -> Mux1/2
  [NR] -> Divide6/2
  Mux/1 -> Divide5/2
  Demux/1 -> PwrInHP/1
  PemH/1 -> Mux9/1
  PemL/1 -> Mux9/2
  Demux/2 -> PwrInLP/1
  Bus Selector2/4 -> Gain3/1  "<NemPsen>"
  Bus Selector2/3 -> Gain2/1  "<NemCsen>"
  Sens/1 -> Bus Selector2/1
  Gain2/1 -> [NC]
  Gain/1 -> [NS]
  Bus Selector2/1 -> Gain/1  "<NemSsen>"
  Bus Selector2/2 -> Gain1/1  "<NemRsen>"
  Gain3/1 -> [NP]
  Gain1/1 -> [NR]
  Sum of Elements/1 -> [PS]
  Sum of Elements1/1 -> [PR]
  Sum of Elements2/1 -> [PC]

== system AGTF30SysDyn_PExPIn/Control System/Steady State EM Power ==
  note: Electric Power Transfer (EPT)
  note: Boost Power
  note: Power Extraction
  Alt : Inport
  MN : Inport  Port=2
  PExAC : Inport  Port=3
  Boost : Inport  Port=4
  EPT : Inport  Port=5
  N1cN : Inport  Port=6
  Sens : Inport  Port=7
  Bus Selector9 : BusSelector  OutputSignals=SOC
  Constant : Constant  Value=MWS.Cntrl.Hyb.Boost.MaxPwr
  Constant1 : Constant  Value=MWS.Cntrl.Hyb.EPT.MaxPwr
  Constant2 : Constant  Value=MWS.In.Options.HybridConfig
  Constant4 : Constant  Value=0
  Demux : Demux  Outputs=2
  Divide : Product  Inputs=****
  Divide1 : Product  Inputs=***
  Divide2 : Product  Inputs=**
  Divide3 : Product  Inputs=**
  Gain1 : Gain  Gain=-1
  Gain2 : Gain  Gain=-1
  Gain3 : Gain  Gain=-1
  HP Pwr Frac Lookup Table : Lookup_n-D  NumberOfTableDimensions=3  BreakpointsForDimension1=MWS.Cntrl.Hyb.PEx.PwrSplitSched.NcFanN_vec  BreakpointsForDimension2=MWS.Cntrl.Hyb.PEx.PwrSplitSched.Alt_vec  BreakpointsForDimension3=MWS.Cntrl.Hyb.PEx.PwrSplitSched.MN_vec  Table=MWS.Cntrl.Hyb.PEx.PwrSplitSched.PwrFracHP_array  InternalRulePriority=Speed  RndMeth=Simplest
      settings: InputPortMap=u0,u1,u2
  Multiport Switch : MultiPortSwitch  SaturateOnIntegerOverflow=off  InputSameDT=off
  Mux : Mux  Inputs=2
  Mux1 : Mux  Inputs=2
  Mux2 : Mux  Inputs=2
  PwrFrac Lookup Table : Lookup_n-D  NumberOfTableDimensions=1  BreakpointsForDimension1=MWS.Cntrl.Hyb.Boost.PwrFracSched.NcFanN_vec  BreakpointsForDimension2=MWS.Cntrl.PHpwr.Sched.MN_vec  Table=MWS.Cntrl.Hyb.Boost.PwrFracSched.PwrFrac_vec  InternalRulePriority=Speed  RndMeth=Simplest
  Rate Limiter : RateLimiter  RisingSlewLimit=MWS.Cntrl.Hyb.Boost.RL  FallingSlewLimit=-MWS.Cntrl.Hyb.Boost.RL  SampleTimeMode=inherited
  Rate Limiter1 : RateLimiter  RisingSlewLimit=MWS.Cntrl.Hyb.EPT.RL  FallingSlewLimit=-MWS.Cntrl.Hyb.EPT.RL  SampleTimeMode=inherited
  Sum2 : Sum  Inputs=|+-
  Sum5 : Sum  Inputs=|+-
  Total PEx Lookup Table : Lookup_n-D  NumberOfTableDimensions=3  BreakpointsForDimension1=MWS.Cntrl.Hyb.PEx.PExSched.NcFanN_vec  BreakpointsForDimension2=MWS.Cntrl.Hyb.PEx.PExSched.Alt_vec  BreakpointsForDimension3=MWS.Cntrl.Hyb.PEx.PExSched.MN_vec  Table=MWS.Cntrl.Hyb.PEx.PExSched.Pwr_array  InternalRulePriority=Speed  RndMeth=Simplest
      settings: InputPortMap=u0,u1,u2
  phiN1cN Lookup Table1 : Lookup_n-D  NumberOfTableDimensions=1  BreakpointsForDimension1=MWS.Cntrl.Hyb.EPT.Sched.N1cN_vec  BreakpointsForDimension2=MWS.Cntrl.PHpwr.Sched.MN_vec  Table=MWS.Cntrl.Hyb.EPT.Sched.phiPwrLvl_vec  InternalRulePriority=Speed  RndMeth=Simplest
  phiSOC Lookup Table : Lookup_n-D  NumberOfTableDimensions=1  BreakpointsForDimension1=MWS.Cntrl.Hyb.Boost.phiSOCSched.SOC_vec  BreakpointsForDimension2=MWS.Cntrl.PHpwr.Sched.MN_vec  Table=MWS.Cntrl.Hyb.Boost.phiSOCSched.phiSOC_vec  InternalRulePriority=Speed  RndMeth=Simplest
  PwrInLP_Base : Outport
  PwrInHP_Base : Outport  Port=2
  PwrEPT : Outport  Port=3
  phiEPT : Outport  Port=4
  phiBoost : Outport  Port=5
  wires:
  Constant/1 -> Divide/3  "MaxPwr"
  MN/1 -> [MN]
  [SOC] -> phiSOC Lookup Table/1
  phiSOC Lookup Table/1 -> Divide3/2, Divide/2  "phiSOC"
  [BoostToggle] -> Rate Limiter/1
  Alt/1 -> [Alt]
  PwrFrac Lookup Table/1 -> Divide/4  "PwrFrac"
  Sens/1 -> Bus Selector9/1
  Rate Limiter/1 -> Divide3/1, Divide/1  "phiTS"
  [N1cN] -> PwrFrac Lookup Table/1
  N1cN/1 -> [N1cN]
  Boost/1 -> [BoostToggle]
  Divide/1 -> [PwrB]  "P_Boost"
  [EPTToggle] -> Rate Limiter1/1
  [N1cN] -> phiN1cN Lookup Table1/1
  phiN1cN Lookup Table1/1 -> Divide1/2  "phiPwrLvl"
  Rate Limiter1/1 -> phiEPT/1, Divide1/1  "phiTS"
  [PwrB] -> Mux/1
  [PwrPEx_HP] -> Sum2/1
  Sum2/1 -> Mux2/2
  [PwrPEx_LP] -> Mux2/1
  Mux1/1 -> Multiport Switch/2
  Mux/1 -> Multiport Switch/3
  Mux2/1 -> Multiport Switch/4
  Constant2/1 -> Multiport Switch/1
  [PExAC] -> Gain1/1
  Gain1/1 -> Mux1/2
  Multiport Switch/1 -> Demux/1
  Demux/1 -> PwrInLP_Base/1
  Demux/2 -> PwrInHP_Base/1
  [PExAC] -> Gain3/1
  [PExAC] -> Sum2/2
  Gain3/1 -> Mux/2
  [N1cN] -> HP Pwr Frac Lookup Table/1, Total PEx Lookup Table/1
  [Alt] -> HP Pwr Frac Lookup Table/2, Total PEx Lookup Table/2
  [MN] -> HP Pwr Frac Lookup Table/3, Total PEx Lookup Table/3
  Total PEx Lookup Table/1 -> Gain2/1  "Total Pwr"
  HP Pwr Frac Lookup Table/1 -> Divide2/2  "HP Pwr Frac"
  Divide2/1 -> [PwrPEx_HP], Sum5/2
  Gain2/1 -> Divide2/1, Sum5/1
  Sum5/1 -> [PwrPEx_LP]
  EPT/1 -> [EPTToggle]
  PExAC/1 -> [PExAC]
  Divide1/1 -> [PwrEPT]  "PwrEPT"
  Constant1/1 -> Divide1/3
  Bus Selector9/1 -> [SOC]  "<SOC>"
  [PwrEPT] -> PwrEPT/1
  Constant4/1 -> Mux1/1
  Divide3/1 -> phiBoost/1  "phiBoost"

== system AGTF30SysDyn_PExPIn/Control System/VAFN Controller ==
  CntrlInput : Inport
  PreLookup : Inport  Port=2
  Bus Selector1 : BusSelector  OutputSignals=ManualOp.VAFNMan,ManualOp.VAFNManEn
  Bus Selector2 : BusSelector  OutputSignals=k_PL,f_PL,k_Alt,f_Alt,k_MN,f_MN,k_PwrInLP,f_PwrInLP,k_PwrInHP,f_PwrInHP
  Interpolation Using Prelookup : Interpolation_n-D  NumberOfTableDimensions=5  Table=MWS.Cntrl.VAFN.Sched.VAFN_array  InternalRulePriority=Speed
      settings: InputPortMap=u0,u1,u2,u3,u4,u5,u6,u7,u8,u9
  Switch : Switch  Criteria=u2 > Threshold  SaturateOnIntegerOverflow=off  InputSameDT=off
  VAFN : Outport  VectorParamsAs1DForOutWhenUnconnected=off
  wires:
  Bus Selector2/1 -> Interpolation Using Prelookup/1  "<k_PL>"
  Bus Selector2/10 -> Interpolation Using Prelookup/10  "<f_PwrInHP>"
  Bus Selector2/3 -> Interpolation Using Prelookup/3  "<k_Alt>"
  Bus Selector2/6 -> Interpolation Using Prelookup/6  "<f_MN>"
  Bus Selector2/9 -> Interpolation Using Prelookup/9  "<k_PwrInHP>"
  PreLookup/1 -> Bus Selector2/1
  Interpolation Using Prelookup/1 -> [VAFN_Sched]
  Bus Selector2/5 -> Interpolation Using Prelookup/5  "<k_MN>"
  Bus Selector2/4 -> Interpolation Using Prelookup/4  "<f_Alt>"
  Switch/1 -> VAFN/1
  CntrlInput/1 -> Bus Selector1/1
  Bus Selector1/1 -> [VAFNMan]  "<VAFNMan>"
  Bus Selector1/2 -> [VAFNManEn]  "<VAFNManEn>"
  [VAFNManEn] -> Switch/2
  [VAFNMan] -> Switch/1
  [VAFN_Sched] -> Switch/3
  Bus Selector2/7 -> Interpolation Using Prelookup/7  "<k_PwrInLP>"
  Bus Selector2/8 -> Interpolation Using Prelookup/8  "<f_PwrInLP>"
  Bus Selector2/2 -> Interpolation Using Prelookup/2  "<f_PL>"

== system AGTF30SysDyn_PExPIn/Control System/VBV Controller ==
  CntrlInput : Inport
  PreLookup : Inport  Port=2
  Bus Selector1 : BusSelector  OutputSignals=ManualOp.VBVMan,ManualOp.VBVManEn
  Bus Selector2 : BusSelector  OutputSignals=k_PL,f_PL,k_Alt,f_Alt,k_MN,f_MN,k_PwrInLP,f_PwrInLP,k_PwrInHP,f_PwrInHP
  Interpolation Using Prelookup : Interpolation_n-D  NumberOfTableDimensions=5  Table=MWS.Cntrl.VBV.Sched.VBV_array  InternalRulePriority=Speed
      settings: InputPortMap=u0,u1,u2,u3,u4,u5,u6,u7,u8,u9
  Switch : Switch  Criteria=u2 > Threshold  SaturateOnIntegerOverflow=off  InputSameDT=off
  VBV : Outport  VectorParamsAs1DForOutWhenUnconnected=off
  wires:
  CntrlInput/1 -> Bus Selector1/1
  Bus Selector1/1 -> [VBVMan]  "<VBVMan>"
  Bus Selector1/2 -> [VBVManEn]  "<VBVManEn>"
  [VBVManEn] -> Switch/2
  [VBVMan] -> Switch/1
  [VBV_Sched] -> Switch/3
  Switch/1 -> VBV/1
  PreLookup/1 -> Bus Selector2/1
  Bus Selector2/3 -> Interpolation Using Prelookup/3  "<k_Alt>"
  Bus Selector2/4 -> Interpolation Using Prelookup/4  "<f_Alt>"
  Bus Selector2/5 -> Interpolation Using Prelookup/5  "<k_MN>"
  Bus Selector2/6 -> Interpolation Using Prelookup/6  "<f_MN>"
  Bus Selector2/9 -> Interpolation Using Prelookup/9  "<k_PwrInHP>"
  Bus Selector2/10 -> Interpolation Using Prelookup/10  "<f_PwrInHP>"
  Interpolation Using Prelookup/1 -> [VBV_Sched]
  Bus Selector2/1 -> Interpolation Using Prelookup/1  "<k_PL>"
  Bus Selector2/2 -> Interpolation Using Prelookup/2  "<f_PL>"
  Bus Selector2/7 -> Interpolation Using Prelookup/7  "<k_PwrInLP>"
  Bus Selector2/8 -> Interpolation Using Prelookup/8  "<f_PwrInLP>"

== system AGTF30SysDyn_PExPIn/Control System/Wf Controller ==
  Calc : Inport
  Sens : Inport  Port=2
  CntrlInput : Inport  Port=3
  Prelookup : Inport  Port=4
  Wfmin : Inport  Port=5
  Wfmax : Inport  Port=6
  phiEPT : Inport  Port=7
  phiBoost : Inport  Port=8
  N1cN : Inport  Port=9
  Bus Selector : BusSelector  OutputSignals=N.N1sen,N.N3sen,P.Ps3sen,T.T2sen,T.T3sen,T.T4sen,T.T45sen
  Bus Selector1 : BusSelector  OutputSignals=ManualOp.WfMan,ManualOp.WfManEn,ManualOp.N1cMan,ManualOp.N1cManEn
  Bus Selector2 : BusSelector  OutputSignals=Alt,MN
  Controller : Subsystem
  Corrected Speed Calc : Subsystem
  Switch : Switch  Criteria=u2 > Threshold  SaturateOnIntegerOverflow=off  InputSameDT=off
  Wf : Outport  VectorParamsAs1DForOutWhenUnconnected=off
  RegNum : Outport  Port=2  VectorParamsAs1DForOutWhenUnconnected=off
  SPs : Outport  Port=3  VectorParamsAs1DForOutWhenUnconnected=off
  N1cErr : Outport  Port=4  VectorParamsAs1DForOutWhenUnconnected=off
  wires:
  [WfMan] -> Switch/1
  [WfManEn] -> Switch/2
  Bus Selector1/2 -> [WfManEn]  "<WfManEn>"
  Bus Selector1/1 -> [WfMan]  "<WfMan>"
  Sens/1 -> Bus Selector/1
  CntrlInput/1 -> Bus Selector1/1
  Bus Selector/4 -> [T2]  "<T2sen>"
  Bus Selector/3 -> [Ps3]  "<Ps3sen>"
  Bus Selector/5 -> [T3]  "<T3sen>"
  Bus Selector/6 -> [T4]  "<T4sen>"
  Switch/1 -> Wf/1
  [N1] -> Corrected Speed Calc/1(N)
  [T2] -> Corrected Speed Calc/2(T)
  Corrected Speed Calc/1(Nc) -> [NcFan]
  [Prelookup] -> Controller/1(Prelookup)
  [NcFan] -> Controller/4(N1c)
  [N3] -> Controller/6(N3)
  [Ps3] -> Controller/7(Ps3)
  [T3] -> Controller/8(T3)
  [T4] -> Controller/9(T4)
  [N1] -> Controller/5(N1)
  Bus Selector/7 -> [T45]  "<T45sen>"
  [Wfdmd] -> Switch/3
  Controller/1(Wfdmd) -> [Wfdmd]
  Controller/2(RegNum) -> [RegNum]
  Controller/3(SPs) -> [SPs]
  [SPs] -> SPs/1
  [RegNum] -> RegNum/1
  Bus Selector1/3 -> [N1cMan]  "<N1cMan>"
  Bus Selector1/4 -> [N1cManEn]  "<N1cManEn>"
  [N1cMan] -> Controller/12(NcFanMan)
  [N1cManEn] -> Controller/11(NcFanManEn)
  Prelookup/1 -> [Prelookup]
  Calc/1 -> Bus Selector2/1
  Bus Selector2/1 -> [Alt]  "<Alt>"
  [Alt] -> Controller/2(Alt)
  Wfmin/1 -> [Wfmin]
  Wfmax/1 -> [Wfmax]
  [Wfmin] -> Controller/13(Wfmin)
  [Wfmax] -> Controller/14(Wfmax)
  Bus Selector/1 -> [N1]  "<N1sen>"
  Bus Selector/2 -> [N3]  "<N3sen>"
  [T45] -> Controller/10(T45)
  Controller/4(N1cErr) -> [N1cErr]
  [N1cErr] -> N1cErr/1
  Bus Selector2/2 -> [MN]  "<MN>"
  phiEPT/1 -> [phiEPT]
  phiBoost/1 -> [phiBoost]
  [MN] -> Controller/3(MN)
  [phiEPT] -> Controller/15(phiEPT)
  [phiBoost] -> Controller/16(phiBoost)
  N1cN/1 -> [N1cN]
  [N1cN] -> Controller/17(N1cN)

== system AGTF30SysDyn_PExPIn/EngineSystem/EngineDW ==
  note: Independent/Dependent Solver
  note: Engine Model Call
  EngSysInp : Inport
  Effectors : Inport  Port=2
  N2 : Inport  Port=3
  N3 : Inport  Port=4
  Bus Creator1 : BusCreator  Inputs=3
  Bus Selector : BusSelector  OutputSignals=Alt,dT,MN
  Bus Selector1 : BusSelector  OutputSignals=Wfact,VAFNact,VBVact
  Bus Selector2 : BusSelector  OutputSignals=EngInp
  Bus Selector3 : BusSelector  OutputSignals=TrqEML,TrqEMH,TrqEMS,TrqEMR,TrqEMC,TrqEMP
  Constant : Constant
  Demux : Demux  Outputs=2
  Engine Model : ModelReference  ModelNameDialog=AGTF30_eng.slx  SimulationMode=Normal  ModelReferenceVersion=18.1
  Iterative NR Solver w JacobianCalc : Lib_Solve_IterNRSolverJC_TMATS/Iterative NR Solver w JacobianCalc  SJac_Per_M=MWS.Init.Solver.Dyn.JPer  SNR_IC_M=MWS.Init.Solver.Dyn.IC  SNR_DX_M=MWS.Init.Solver.Dyn.dX  SNR_Mx_M=100000  SNR_Mn_M=0.0001  SJacobianAttempts_M=MWS.Init.Solver.Dyn.NRA  Cond_Limits_M=MWS.Init.Solver.Dyn.Lim
  Mux1 : Mux  Inputs=14
  Mux2 : Mux  Inputs=2
  Signal Conversion : SignalConversion  OverrideOpt=off
  Signal Conversion1 : SignalConversion  OverrideOpt=off
  Subsystem : Subsystem
  Terminator : Terminator
  While Iterator : WhileIterator  MaxIters=MWS.Init.Max_IterDyn  WhileBlockType=do-while  ShowIterationPort=on
  EngOut : Outport
  Solver : Outport  Port=2
  N2dot : Outport  Port=3
  N3dot : Outport  Port=4
  wires:
  Engine Model/1 -> EngOut/1  "EngBus"
  Mux1/1 -> Engine Model/1
  EngSysInp/1 -> Bus Selector2/1, Subsystem/1(SysIn)
  Effectors/1 -> Bus Selector3/1, Bus Selector1/1
  Constant/1 -> Iterative NR Solver w JacobianCalc/2
  Iterative NR Solver w JacobianCalc/2 -> Engine Model/2, [Indep]  "Independents"
  Engine Model/3 -> Iterative NR Solver w JacobianCalc/3, [Dep]  "Dependents"
  While Iterator/1 -> [Iterations], Iterative NR Solver w JacobianCalc/1
  Iterative NR Solver w JacobianCalc/1 -> While Iterator/1
  Engine Model/2 -> Demux/1
  Mux2/1 -> Subsystem/2(N), Engine Model/3
  Iterative NR Solver w JacobianCalc/3 -> Terminator/1
  N2/1 -> Mux2/1
  N3/1 -> Mux2/2
  Demux/1 -> N2dot/1
  Demux/2 -> N3dot/1
  Bus Selector/1 -> Mux1/1  "<Alt>"
  Bus Selector/2 -> Mux1/2  "<dT>"
  Bus Selector/3 -> Mux1/3  "<MN>"
  Bus Selector1/3 -> Mux1/6  "<VBVact>"
  Bus Selector1/1 -> Mux1/4  "<Wfact>"
  [Iterations] -> Bus Creator1/1  "Iterations"
  Bus Creator1/1 -> Solver/1  "Solver"
  [Dep] -> Signal Conversion1/1
  [Indep] -> Signal Conversion/1
  Signal Conversion/1 -> Bus Creator1/3  "Independents"
  Signal Conversion1/1 -> Bus Creator1/2  "Dependents"
  Bus Selector1/2 -> Mux1/5  "<VAFNact>"
  Bus Selector2/1 -> Bus Selector/1  "<EngInp>"
  Subsystem/1(TrqInLP) -> Mux1/7
  Subsystem/2(TrqInHP) -> Mux1/8
  Bus Selector3/1 -> Mux1/9  "<TrqEML>"
  Bus Selector3/2 -> Mux1/10  "<TrqEMH>"
  Bus Selector3/3 -> Mux1/11  "<TrqEMS>"
  Bus Selector3/4 -> Mux1/12  "<TrqEMR>"
  Bus Selector3/5 -> Mux1/13  "<TrqEMC>"
  Bus Selector3/6 -> Mux1/14  "<TrqEMP>"

== system AGTF30SysDyn_PExPIn/EngineSystem/Power System ==
  Load [hp] : Inport
  Nem : Inport  Port=2
  TrqEM : Inport  Port=3
  Bus Creator : BusCreator  Inputs=2
  Bus Creator1 : BusCreator  Inputs=7
  Bus Selector : BusSelector  OutputSignals=GBData.DEM.Nem,GBData.PGB.Nem
  Bus Selector1 : BusSelector  OutputSignals=TrqEML,TrqEMH,TrqEMS,TrqEMR,TrqEMC,TrqEMP
  Demux : Demux  Outputs=2
  Demux1 : Demux
  Electrical Power System : Subsystem
  PwrSysOut : Outport
  wires:
  Demux1/4 -> [NemP]
  Bus Selector1/3 -> [TrqEMS]  "<TrqEMS>"
  Electrical Power System/3(Out_SEMbranch) -> Bus Creator1/3  "EMSbranch"
  Bus Selector1/4 -> [TrqEMR]  "<TrqEMR>"
  [NemP] -> Electrical Power System/11(NemP [rpm])
  Bus Selector/2 -> Demux1/1  "<Nem>"
  [TrqEMH] -> Electrical Power System/4(TrqEMH [ft-lb])
  [TrqEMS] -> Electrical Power System/6(TrqEMS [ft-lb])
  Demux/1 -> [NemL]
  [NemC] -> Electrical Power System/9(NemC [rpm])
  Bus Selector1/2 -> [TrqEMH]  "<TrqEMH>"
  [NemS] -> Electrical Power System/5(NemS [rpm])
  Bus Selector1/1 -> [TrqEML]  "<TrqEML>"
  Load [hp]/1 -> Electrical Power System/13(Load [hp])
  [TrqEMR] -> Electrical Power System/8(TrqEMR [ft-lb])
  Nem/1 -> Bus Selector/1
  Demux1/3 -> [NemC]
  Bus Selector1/5 -> [TrqEMC]  "<TrqEMC>"
  [TrqEMC] -> Electrical Power System/10(TrqEMC [ft-lb])
  Demux1/1 -> [NemS]
  [NemR] -> Electrical Power System/7(NemR [rpm])
  Bus Selector/1 -> Demux/1  "<Nem>"
  Bus Selector1/6 -> [TrqEMP]  "<TrqEMP>"
  Electrical Power System/1(Out_LPEMbranch) -> Bus Creator1/1  "EMLbranch"
  [NemH] -> Electrical Power System/3(NemH [rpm])
  Demux/2 -> [NemH]
  [TrqEMP] -> Electrical Power System/12(TrqEMP [ft-lb])
  Electrical Power System/6(Out_PEMbranch) -> Bus Creator1/6  "EMPbranch"
  [NemL] -> Electrical Power System/1(NemL [rpm])
  [TrqEML] -> Electrical Power System/2(TrqEML [ft-lb])
  Demux1/2 -> [NemR]
  Electrical Power System/4(Out_REMbranch) -> Bus Creator1/4  "EMRbranch"
  Bus Creator1/1 -> Bus Creator/1  "Pwrs"
  Electrical Power System/5(Out_CEMbranch) -> Bus Creator1/5  "EMCbranch"
  Electrical Power System/7(Out_SupplySys) -> Bus Creator1/7  "Supplybranch"
  Electrical Power System/2(Out_HPEMbranch) -> Bus Creator1/2  "EMHbranch"
  TrqEM/1 -> Bus Selector1/1
  Bus Creator/1 -> PwrSysOut/1
  Electrical Power System/8(SoC [%]) -> Bus Creator/2  "SOC"

== system AGTF30SysDyn_PExPIn/Actuators/Carrier Electric Machine/Power [hp] to Torque [ft-lb] ==
  N : Inport
  P : Inport  Port=2
  Divide2 : Product  Inputs=/*
  Gain : Gain  Gain=5252.113
  Trq : Outport  VectorParamsAs1DForOutWhenUnconnected=off
  wires:
  P/1 -> Gain/1
  Gain/1 -> Divide2/2
  N/1 -> Divide2/1
  Divide2/1 -> Trq/1

== system AGTF30SysDyn_PExPIn/Actuators/HPS Electric Machine/Power [hp] to Torque [ft-lb] ==
  N : Inport
  P : Inport  Port=2
  Divide2 : Product  Inputs=/*
  Gain : Gain  Gain=5252.113
  Trq : Outport  VectorParamsAs1DForOutWhenUnconnected=off
  wires:
  P/1 -> Gain/1
  Gain/1 -> Divide2/2
  N/1 -> Divide2/1
  Divide2/1 -> Trq/1

== system AGTF30SysDyn_PExPIn/Actuators/LPS Electric Machine/Power [hp] to Torque [ft-lb] ==
  N : Inport
  P : Inport  Port=2
  Divide2 : Product  Inputs=/*
  Gain : Gain  Gain=5252.113
  Trq : Outport  VectorParamsAs1DForOutWhenUnconnected=off
  wires:
  P/1 -> Gain/1
  Gain/1 -> Divide2/2
  N/1 -> Divide2/1
  Divide2/1 -> Trq/1

== system AGTF30SysDyn_PExPIn/Actuators/Planet Gear Electric Machine/Power [hp] to Torque [ft-lb] ==
  N : Inport
  P : Inport  Port=2
  Divide2 : Product  Inputs=/*
  Gain : Gain  Gain=5252.113
  Trq : Outport  VectorParamsAs1DForOutWhenUnconnected=off
  wires:
  P/1 -> Gain/1
  Gain/1 -> Divide2/2
  N/1 -> Divide2/1
  Divide2/1 -> Trq/1

== system AGTF30SysDyn_PExPIn/Actuators/Ring Gear Electric Machine/Power [hp] to Torque [ft-lb] ==
  N : Inport
  P : Inport  Port=2
  Divide2 : Product  Inputs=/*
  Gain : Gain  Gain=5252.113
  Trq : Outport  VectorParamsAs1DForOutWhenUnconnected=off
  wires:
  P/1 -> Gain/1
  Gain/1 -> Divide2/2
  N/1 -> Divide2/1
  Divide2/1 -> Trq/1

== system AGTF30SysDyn_PExPIn/Actuators/Sun Gear Electric Machine/Power [hp] to Torque [ft-lb] ==
  N : Inport
  P : Inport  Port=2
  Divide2 : Product  Inputs=/*
  Gain : Gain  Gain=5252.113
  Trq : Outport  VectorParamsAs1DForOutWhenUnconnected=off
  wires:
  P/1 -> Gain/1
  Gain/1 -> Divide2/2
  N/1 -> Divide2/1
  Divide2/1 -> Trq/1

== system AGTF30SysDyn_PExPIn/Control System/Electric Machine Controllers/EM Controllers ==
  PwrInLPEMNomMan : Inport
  PwrInLPEMNomManEn : Inport  Port=2
  PwrInLPEMOffNomMan : Inport  Port=3
  PwrInLPEMOffNomManEn : Inport  Port=4
  PwrInHPEMNomMan : Inport  Port=5
  PwrInHPEMNomManEn : Inport  Port=6
  PwrInHPEMOffNomMan : Inport  Port=7
  PwrInHPEMOffNomManEn : Inport  Port=8
  PwrInSEMNomMan : Inport  Port=9
  PwrInSEMNomManEn : Inport  Port=10
  PwrInSEMOffNomMan : Inport  Port=11
  PwrInSEMOffNomManEn : Inport  Port=12
  PwrInREMNomMan : Inport  Port=13
  PwrInREMNomManEn : Inport  Port=14
  PwrInREMOffNomMan : Inport  Port=15
  PwrInREMOffNomManEn : Inport  Port=16
  PwrInCEMNomMan : Inport  Port=17
  PwrInCEMNomManEn : Inport  Port=18
  PwrInCEMOffNomMan : Inport  Port=19
  PwrInCEMOffNomManEn : Inport  Port=20
  PwrInPEMNomMan : Inport  Port=21
  PwrInPEMNomManEn : Inport  Port=22
  PwrInPEMOffNomMan : Inport  Port=23
  PwrInPEMOffNomManEn : Inport  Port=24
  PwrInLP_Base : Inport  Port=25
  PwrInHP_Base : Inport  Port=26
  NemL : Inport  Port=27
  NemH : Inport  Port=28
  NemS : Inport  Port=29
  NemR : Inport  Port=30
  NemC : Inport  Port=31
  NemP : Inport  Port=32
  PwrEPT : Inport  Port=33
  PwrInAccel_TEEM : Inport  Port=34
  PwrExAccel_TEEM : Inport  Port=35
  PwrXDecel_TEEM : Inport  Port=36
  PwrCharge : Inport  Port=37
  PExAC : Inport  Port=38
  PwrSys : Inport  Port=39
  N1cErrN : Inport  Port=40
  DEM Control : Subsystem  VariantControl=MWS.In.Options.EngineEMInt == 1
  PGB EM Control : Subsystem  VariantControl=MWS.In.Options.EngineEMInt == 2
  PwrEML : Outport
  TrqEML : Outport  Port=2
  PwrEMH : Outport  Port=3
  TrqEMH : Outport  Port=4
  PwrEMS : Outport  Port=5
  TrqEMS : Outport  Port=6
  PwrEMR : Outport  Port=7
  TrqEMR : Outport  Port=8
  PwrEMC : Outport  Port=9
  TrqEMC : Outport  Port=10
  PwrEMP : Outport  Port=11
  TrqEMP : Outport  Port=12
  PwrLoad : Outport  Port=13

== system AGTF30SysDyn_PExPIn/Control System/Electric Machine Controllers/SOC Controller ==
  note: PICKUP UPDATING SOC CONTROL AND GETTING CORRECT LOAD
      |
      | LOAD SHOULD INCLUDE: PExAC AND PEx FOR PROPULSION.
      | FOR REG AND BOOST, PLOAD SHOULD JUST BE PExAC. FOR
      | PEx, PLOAD CAN BE CALCULATED WITH PWR_BASE.
  note: NOTE: THE SOC CONTROLLER WILL BE LIMITED BY THE EM LIMITATIONS.
      | THIS MEANS WHEN HIGH POWER, CHARGING COULD TAKE LONGER OR NOT OCCUR. HIGH POWER SHOULD TAKE PRIORITY BECAUSE WE DON"T WANT TO LIMIT THE MAXIMUM POWER IN THE EVENTOF A GO-AROUND OR SOME OTHER SAFETY CRITICAL EVENT. WILL FAVOR TAKING POWER FROM THE HP BECAUSE
      | ALL CONFIGURATIONS WILL HAVE AN HP EM.
  note: Postive value representing and power extraction. Must be subtracted later.
  note: RATE LIMIT TO PREVENT ABRUPT CHANGES IN CHARGING POWER.
  note: MAXIMUM CHARGING/DISCHARGING POWER TO LIMIT LARGE SWINGS
  SOC : Inport
  ChargeToggle : Inport  Port=2
  BoostToggle : Inport  Port=3
  N1cErrN : Inport  Port=4
  N1cN : Inport  Port=5
  Abs : Abs  SaturateOnIntegerOverflow=off
  Compare To Constant : simulink/Logic and Bit Operations/Compare To Constant  relop===  const=2  OutDataTypeStr=boolean
  Compare To Constant1 : simulink/Logic and Bit Operations/Compare To Constant  relop=<  const=0.5  OutDataTypeStr=boolean
  Compare To Constant2 : simulink/Logic and Bit Operations/Compare To Constant  relop===  const=0  OutDataTypeStr=boolean
  Constant1 : Constant  Value=0
  Constant2 : Constant  Value=MWS.Cntrl.SOCReg.PwrCharge.SOC_targ
  Constant3 : Constant  Value=MWS.Cntrl.SOCReg.PwrCharge.Kp
  Constant4 : Constant  Value=MWS.Cntrl.SOCReg.PwrCharge.Ki
  Constant5 : Constant  Value=0
  Constant6 : Constant  Value=0
  Constant7 : Constant  Value=MWS.In.Options.HybridConfig
  Divide1 : Product  Inputs=**
  Divide2 : Product  Inputs=**
  Divide3 : Product  Inputs=**
  Logical Operator : Logic  Operator=OR  AllPortsSameDT=off  OutDataTypeStr=boolean
  Logical Operator1 : Logic  AllPortsSameDT=off  OutDataTypeStr=boolean
  MinMax : MinMax
  Mux : Mux  Inputs=2
  Pmax Charge : Lookup_n-D  NumberOfTableDimensions=1  BreakpointsForDimension1=MWS.Cntrl.SOCReg.PwrCharge.N1cN_vec  Table=MWS.Cntrl.SOCReg.PwrCharge.Pmax_vec  ExtrapMethod=Clip  InternalRulePriority=Speed  RndMeth=Simplest
  Rate Limiter : RateLimiter  RisingSlewLimit=MWS.Cntrl.SOCReg.PwrRateLim  FallingSlewLimit=-MWS.Cntrl.SOCReg.PwrRateLim  SampleTimeMode=inherited
  Set Point Controller (PI) : Subsystem  mask(T-MATS: Set Point Controller (PI)){PI_IC_M=0, WGain_M=MWS.Cntrl.SOCReg.PwrCharge.Kiwp, Ts_M=MWS.In.Ts}
      mask prompts: PI_IC_M "PI_IC_M - PI initial condition"; WGain_M "WGain_M - Windup protection gain"; Ts_M "Ts_M - Sample time"
      mask help: This block contains a PI controller with anti-windup protection. Gains, Kp and Ki, are define external to the block.
      mask Help: web(which('Control_TMATS_SPCPI.html'),'-helpbrowser')
  Sign : Signum
  Sum : Sum  Inputs=|+-
  Sum1 : Sum  Inputs=|++
  Switch : Switch  Criteria=u2 > Threshold  SaturateOnIntegerOverflow=off  InputSameDT=off
  Terminator : Terminator
  Transient Deactivation : Lookup_n-D  NumberOfTableDimensions=1  BreakpointsForDimension1=MWS.Cntrl.SOCReg.Activation.N1cErrN_vec  Table=MWS.Cntrl.SOCReg.Activation.Param_vec  ExtrapMethod=Clip  InternalRulePriority=Speed  RndMeth=Simplest
  PwrCharge : Outport
  wires:
  Logical Operator/1 -> Compare To Constant2/1, Switch/2
  Switch/1 -> Rate Limiter/1
  Constant1/1 -> Switch/1
  Rate Limiter/1 -> Set Point Controller (PI)/3(Eff_dmd), PwrCharge/1
  Constant2/1 -> Sum/1
  Constant3/1 -> Set Point Controller (PI)/4(Kp)
  Constant4/1 -> Set Point Controller (PI)/5(Ki)
  Constant5/1 -> Set Point Controller (PI)/6(Man_En)
  Constant6/1 -> Set Point Controller (PI)/7(Eff_Man)
  Set Point Controller (PI)/2(Active) -> Terminator/1
  Sum/1 -> Divide1/1
  Sum1/1 -> Set Point Controller (PI)/1(Input_req)
  SOC/1 -> Sum1/2, Sum/2, Set Point Controller (PI)/2(Input_sensed)
  Divide1/1 -> Sum1/1
  N1cErrN/1 -> Transient Deactivation/1
  Transient Deactivation/1 -> Divide3/1
  Set Point Controller (PI)/1(Eff_req) -> Divide3/2
  Constant7/1 -> Compare To Constant/1
  Compare To Constant/1 -> Logical Operator1/2
  ChargeToggle/1 -> Compare To Constant1/1
  Logical Operator1/1 -> Logical Operator/2
  BoostToggle/1 -> Logical Operator1/1
  N1cN/1 -> Pmax Charge/1
  Divide3/1 -> Sign/1, Abs/1
  Divide2/1 -> Switch/3
  Pmax Charge/1 -> Mux/2
  Mux/1 -> MinMax/1
  Abs/1 -> Mux/1
  Sign/1 -> Divide2/1
  Compare To Constant1/1 -> Logical Operator/1
  Compare To Constant2/1 -> Divide1/2
  MinMax/1 -> Divide2/2
